simulink model "diploms"  (R2018b)
settings: Solver=VariableStepAuto  StartTime=0.0  StopTime=50  RelTol=1e-3
settings Model: Creator=Seaking  LastModifiedBy=shevc
settings DebuggingCC: LibraryContextMissingDiagnostic=none
settings SFSimCC: SimUseLocalCustomCode=off
settings RTWCC: RTWUseLocalCustomCode=off

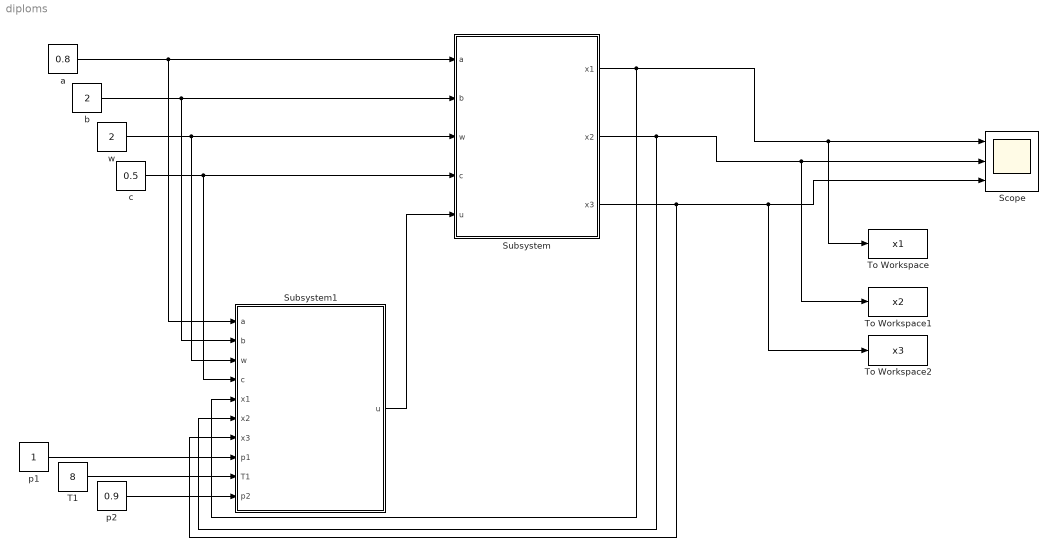
== system diploms ==
  Scope : Scope  NumInputPorts=3
  Subsystem : Subsystem
  Subsystem1 : Subsystem
  T1 : Constant  Value=8
  To Workspace : ToWorkspace  VariableName=x1  SaveFormat=Timeseries  SampleTime=-1
  To Workspace1 : ToWorkspace  VariableName=x2  SaveFormat=Timeseries  SampleTime=-1
  To Workspace2 : ToWorkspace  VariableName=x3  SaveFormat=Timeseries  SampleTime=-1
  a : Constant  Value=0.8
  b : Constant  Value=2
  c : Constant  Value=0.5
  p1 : Constant
  p2 : Constant  Value=0.9
  w : Constant  Value=2
  wires:
  Subsystem/2(x2) -> Subsystem1/6(x2), To Workspace1/1, Scope/2
  Subsystem/3(x3) -> Subsystem1/7(x3), To Workspace2/1, Scope/3
  Subsystem/1(x1) -> Subsystem1/5(x1), To Workspace/1, Scope/1
  a/1 -> Subsystem1/1(a), Subsystem/1(a)
  b/1 -> Subsystem1/2(b), Subsystem/2(b)
  w/1 -> Subsystem1/3(w), Subsystem/3(w)
  c/1 -> Subsystem1/4(c), Subsystem/4(c)
  Subsystem1/1(u) -> Subsystem/5(u)
  p1/1 -> Subsystem1/8(p1)
  T1/1 -> Subsystem1/9(T1)
  p2/1 -> Subsystem1/10(p2)

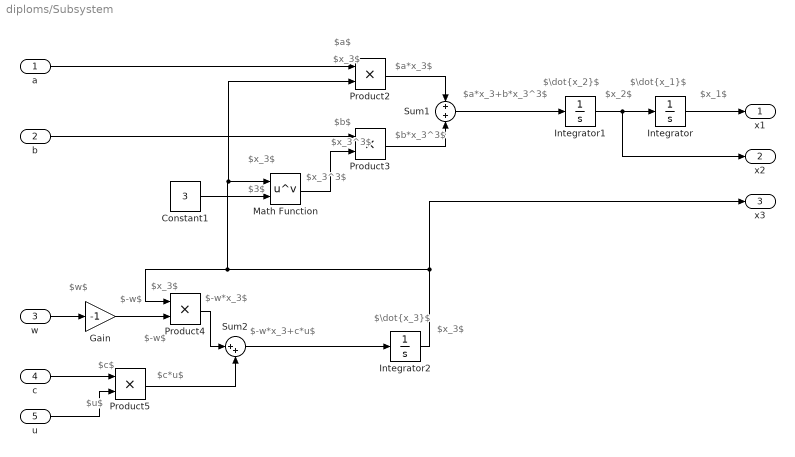
== system diploms/Subsystem ==
  note: $x_3$
  note: $a$
  note: $a*x_3$
  note: $b$
  note: $b*x_3^3$
  note: $\dot{x_2}$
  note: $a*x_3+b*x_3^3$
  note: $x_2$
  note: $\dot{x_1}$
  note: $x_1$
  note: $x_3$
  note: $x_3^3$
  note: $3$
  note: $x_3^3$
  note: $-w*x_3$
  note: $c*u$
  note: $-w$
  note: $w$
  note: $-w*x_3+c*u$
  note: $u$
  note: $x_3$
  note: $-w$
  note: $c$
  note: $\dot{x_3}$
  note: $x_3$
  a : Inport
  b : Inport  Port=2
  w : Inport  Port=3
  c : Inport  Port=4
  u : Inport  Port=5
  Constant1 : Constant  Value=3
  Gain : Gain  Gain=-1
  Integrator : Integrator  InitialCondition=2
  Integrator1 : Integrator  InitialCondition=2
  Integrator2 : Integrator  InitialCondition=2
  Math Function : Math  Operator=pow  SaturateOnIntegerOverflow=on
  Product{2..5} (4 alike) : Product
  Sum1 : Sum
  Sum2 : Sum  Inputs=|++
  x1 : Outport
  x2 : Outport  Port=2
  x3 : Outport  Port=3
  wires:
  a/1 -> Product2/1
  b/1 -> Product3/1
  Integrator1/1 -> x2/1, Integrator/1
  Sum1/1 -> Integrator1/1
  Product2/1 -> Sum1/1
  Product3/1 -> Sum1/2
  Integrator/1 -> x1/1
  Constant1/1 -> Math Function/2
  Math Function/1 -> Product3/2
  Gain/1 -> Product4/2
  Product4/1 -> Sum2/1
  w/1 -> Gain/1
  c/1 -> Product5/1
  Sum2/1 -> Integrator2/1
  Product5/1 -> Sum2/2
  u/1 -> Product5/2
  Integrator2/1 -> x3/1, Product2/2, Math Function/1, Product4/1

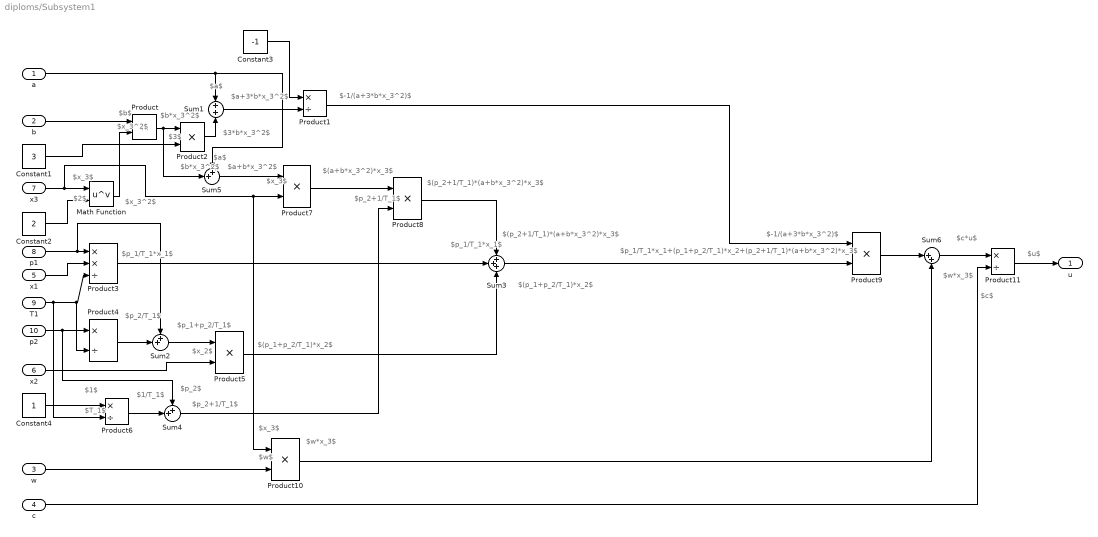
== system diploms/Subsystem1 ==
  note: $x_3$
  note: $x_3^2$
  note: $2$
  note: $b$
  note: $3$
  note: $3*b*x_3^2$
  note: $a$
  note: $a+3*b*x_3^2$
  note: $-1/(a+3*b*x_3^2)$
  note: $p_1/T_1*x_1$
  note: $p_2/T_1$
  note: $p_1+p_2/T_1$
  note: $p_1/T_1*x_1$
  note: $x_2$
  note: $(p_1+p_2/T_1)*x_2$
  note: $(p_1+p_2/T_1)*x_2$
  note: $T_1$
  note: $1$
  note: $1/T_1$
  note: $p_2$
  note: $p_2+1/T_1$
  note: $x_3^2$
  note: $b*x_3^2$
  note: $a$
  note: $b*x_3^2$
  note: $a+b*x_3^2$
  note: $x_3$
  note: $(a+b*x_3^2)*x_3$
  note: $p_2+1/T_1$
  note: $(p_2+1/T_1)*(a+b*x_3^2)*x_3$
  note: $(p_2+1/T_1)*(a+b*x_3^2)*x_3$
  note: $p_1/T_1*x_1+(p_1+p_2/T_1)*x_2+(p_2+1/T_1)*(a+b*x_3^2)*x_3$
  note: $-1/(a+3*b*x_3^2)$
  note: $x_3$
  note: $w$
  note: $w*x_3$
  note: $w*x_3$
  note: $c*u$
  note: $c$
  note: $u$
  a : Inport
  b : Inport  Port=2
  w : Inport  Port=3
  c : Inport  Port=4
  x1 : Inport  Port=5
  x2 : Inport  Port=6
  x3 : Inport  Port=7
  p1 : Inport  Port=8
  T1 : Inport  Port=9
  p2 : Inport  Port=10
  Constant1 : Constant  Value=3
  Constant2 : Constant  Value=2
  Constant3 : Constant  Value=-1
  Constant4 : Constant
  Math Function : Math  Operator=pow  SaturateOnIntegerOverflow=on
  Product{,2,5,7..10} (7 alike) : Product
  Product{1,4,6,11} (4 alike) : Product  Inputs=*/
  Product3 : Product  Inputs=**/
  Sum1 : Sum
  Sum2 : Sum  Inputs=++|
  Sum3 : Sum  Inputs=+++
  Sum4 : Sum  Inputs=++|
  Sum5 : Sum  Inputs=++|
  Sum6 : Sum  Inputs=|++
  u : Outport
  wires:
  x3/1 -> Product10/1, Product7/2, Math Function/1
  Constant2/1 -> Math Function/2
  b/1 -> Product/1
  Product/1 -> Sum5/2, Product2/1
  Product2/1 -> Sum1/2
  a/1 -> Sum5/1, Sum1/1
  Constant3/1 -> Product1/1
  Sum1/1 -> Product1/2
  p1/1 -> Sum2/1, Product3/1
  x1/1 -> Product3/2
  T1/1 -> Product6/2, Product4/2, Product3/3
  p2/1 -> Sum4/1, Product4/1
  Product4/1 -> Sum2/2
  x2/1 -> Product5/2
  Sum2/1 -> Product5/1
  Constant4/1 -> Product6/1
  Product6/1 -> Sum4/2
  Math Function/1 -> Product/2
  Constant1/1 -> Product2/2
  Sum5/1 -> Product7/1
  Product7/1 -> Product8/1
  Sum4/1 -> Product8/2
  Product8/1 -> Sum3/1
  Product5/1 -> Sum3/3
  Product3/1 -> Sum3/2
  Sum3/1 -> Product9/2
  Product1/1 -> Product9/1
  w/1 -> Product10/2
  Product10/1 -> Sum6/2
  Product9/1 -> Sum6/1
  c/1 -> Product11/2
  Sum6/1 -> Product11/1
  Product11/1 -> u/1
